simulink model "ANNModel"  (R2020a)
settings: Solver=VariableStepAuto  StartTime=0.0  StopTime=10.0  RelTol=1e-3
libraries: neural x207
(part 9 of 9)

== system ANNModel/Feed-Forward Neural Network/Layer 4/Delays 1 ==
  "p{4}" : Inport  PortDimensions=50
      mask Display: e = 0.06;c1 = [120 230 180]/255;c2 = ([120 230 180]+0)/(256+128);c3 = ([120 230 180]+128)/(256+128);patch([0 1 1 0],[0 0 1 1],c1);patch([0 1 1 1-e 1-e 0+e],[0 0 1 1-e 0+e 0+e],c2);patch([0 0 1 1-e 0+e 0+e],[0 1 1 1-e 1-e 0+e],c3);plot([0 1 1 0 0],[0 0 1 1 0]);
  mux : Mux  Inputs=1
      mask Display: e = 0.06;c1 = [120 150 230]/255;c2 = ([120 150 230]+0)/383;c3 = ([120 150 230]+128)/383;patch([0 1 1 0],[0 0 1 1],c1);patch([0 1 1 1-e 1-e 0+e],[0 0 1 1-e 0+e 0+e],c2);patch([0 0 1 1-e 0+e 0+e],[0 1 1 1-e 1-e 0+e],c3);plot([0 1 1 0 0],[0 0 1 1 0]);disp('Mux')
  "pd{4,3}" : Outport
      mask Display: e = 0.06;c1 = [120 230 180]/255;c2 = ([120 230 180]+0)/(256+128);c3 = ([120 230 180]+128)/(256+128);patch([0 1 1 0],[0 0 1 1],c1);patch([0 1 1 1-e 1-e 0+e],[0 0 1 1-e 0+e 0+e],c2);patch([0 0 1 1-e 0+e 0+e],[0 1 1 1-e 1-e 0+e],c3);plot([0 1 1 0 0],[0 0 1 1 0]);
  wires:
  "p{4}"/1 -> mux/1
  mux/1 -> "pd{4,3}"/1

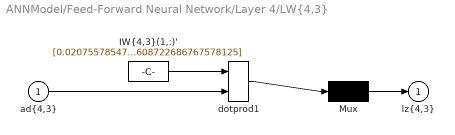
== system ANNModel/Feed-Forward Neural Network/Layer 4/LW{4,3} ==
  "ad{4,3}" : Inport  PortDimensions=50
      mask Display: e = 0.06;c1 = [120 230 180]/255;c2 = ([120 230 180]+0)/(256+128);c3 = ([120 230 180]+128)/(256+128);patch([0 1 1 0],[0 0 1 1],c1);patch([0 1 1 1-e 1-e 0+e],[0 0 1 1-e 0+e 0+e],c2);patch([0 0 1 1-e 0+e 0+e],[0 1 1 1-e 1-e 0+e],c3);plot([0 1 1 0 0],[0 0 1 1 0]);
  "IW{4,3}(1,:)'" : Constant  Value=[0.0207557854765180911649213868486185674555599689483642578125;1.00434019028882648427725143847055733203887939453125;0.420046964791842281083944499187055043876171112060546875;0.75827454684748041291442177680437453091144561767578125;-0.153386070273279495612683831495814956724643707275390625;-0.06371578540448184779787510478854528628289699554443359375;-0.72440112000010870030308751665870659053325653076171875;-0.8242065158490696763493588150595314800739288330078125;-0.04089000128492459307238959809183143079280853271484375;0.86028078276374231325718255902756936848163604736328125;-0.10019412851903232442030144966338411904871463775634765625;-0.376336809495103896683332322936621494591236114501953125;-0.5024897362807383416338780079968273639678955078125;0.88518193199074601817954999205539934337139129638671875;-0.30647566190199648783476504831924103200435638427734375;0.73149803749265374097632275152136571705341339111328125;0.85285320015363785817186226267949678003787994384765625;-0.311341494408280794470300634202430956065654754638671875;-0.455439380404615012931657247463590465486049652099609375;0.05462273658175016699534154440698330290615558624267578125;0.197262875803622839132600574885145761072635650634765625;0.1347505594016246421862348370268591679632663726806640625;-0.76115829763100906202311080051003955304622650146484375;0.1265161997467760535140968158884788863360881805419921875;-0.04427960106054766586947124551443266682326793670654296875;-0.472512782533158703923703569671488367021083831787109375;0.957100988562776588963743051863275468349456787109375;-0.57086502760544111101381758999195881187915802001953125;-0.4866328938014294891445388202555477619171142578125;0.900128017868683460989132072427310049533843994140625;0.484589383654006000679004273479222320020198822021484375;0.019516983704605743443760701438804971985518932342529296875;-0.10407332980398086019757641906835488043725490570068359375;-0.370448078139256342655727394230780191719532012939453125;0.43267137096662444673000891270930878818035125732421875;0.82274142310055886628816779193584807217121124267578125;-0.10999476220115271540844759101673844270408153533935546875;0.54684002679072352126610212508239783346652984619140625;0.1381080156462380081894281147469882853329181671142578125;-0.799569064520076810964610558585263788700103759765625;-0.180259477441625348692610941725433804094791412353515625;-0.33147914761863750410242346333689056336879730224609375;-0.486398147713130002411929808658896945416927337646484375;-0.055642699517251613394730469508431269787251949310302734375;0.1526685461752050887440645965398289263248443603515625;0.7128170456361591078575656865723431110382080078125;-0.94239708871964322778325140461674891412258148193359375;0.468638195744502994433133835627813823521137237548828125;-0.54030322310456602163952766204602085053920745849609375;0.5746343074387774141342788425390608608722686767578125]
      mask Display: e = 0.06;c1 = [120 150 230]/255;c2 = ([120 150 230]+0)/383;c3 = ([120 150 230]+128)/383;patch([0 1 1 0],[0 0 1 1],c1);patch([0 1 1 1-e 1-e 0+e],[0 0 1 1-e 0+e 0+e],c2);patch([0 0 1 1-e 0+e 0+e],[0 1 1 1-e 1-e 0+e],c3);plot([0 1 1 0 0],[0 0 1 1 0]);disp('weights');
  Mux : Mux  Inputs=1
      mask Display: e = 0.06;c1 = [120 150 230]/255;c2 = ([120 150 230]+0)/383;c3 = ([120 150 230]+128)/383;patch([0 1 1 0],[0 0 1 1],c1);patch([0 1 1 1-e 1-e 0+e],[0 0 1 1-e 0+e 0+e],c2);patch([0 0 1 1-e 0+e 0+e],[0 1 1 1-e 1-e 0+e],c3);plot([0 1 1 0 0],[0 0 1 1 0]);disp('Mux');
  dotprod1 : neural/Weight Functions/dotprod
  "lz{4,3}" : Outport
      mask Display: e = 0.06;c1 = [120 230 180]/255;c2 = ([120 230 180]+0)/(256+128);c3 = ([120 230 180]+128)/(256+128);patch([0 1 1 0],[0 0 1 1],c1);patch([0 1 1 1-e 1-e 0+e],[0 0 1 1-e 0+e 0+e],c2);patch([0 0 1 1-e 0+e 0+e],[0 1 1 1-e 1-e 0+e],c3);plot([0 1 1 0 0],[0 0 1 1 0]);
  wires:
  "IW{4,3}(1,:)'"/1 -> dotprod1/1
  "ad{4,3}"/1 -> dotprod1/2
  dotprod1/1 -> Mux/1
  Mux/1 -> "lz{4,3}"/1
